simulink model "W02_surge_control"  (R2024b)
settings: Solver=ode4  StartTime=0  StopTime=T_final  FixedStep=h  RelTol=1e-3
StopFcn:
  | W02_plot;
values from neighbouring files (symbols this model uses):
  animate = 1    [W02_0_setup.m]
  aw_mode = 2    [W02_0_setup.m]
  beta_c = 0    [W02_0_setup.m]
  c_d = 0    [W02_0_setup.m]
  h = 0.02    [W02_0_setup.m]    (also in W02_1_build_pid.m = add_line(sys, [a; via; b]); W02_1_build_surge_control.m = Simulink.Annotation([m '/note']); W02_G_derivative_noise_and_kick.m = lab_fig('W02 G  kick', 1000, 420);  hold on; W02_G_noise_and_kick.m = lab_fig('W02 Exp 2-10c  kick', 1000, 420);  hold on)
  K_aw = 1/T_u    (= 0.907069384191)    [W02_0_setup.m]
  k_neg = cfg.k_neg    [W02_0_setup.m]
  k_pos = cfg.k_pos    [W02_0_setup.m]
  Kd = 0    [W02_0_setup.m]    (also in W02_E_integral.m = 4; W02_I_tuning_by_hand.m = 1)
  Ki = 192.38    [W02_0_setup.m]
  Kp = 102.00    (= 102)    [W02_0_setup.m]    (also in W02_D_derivative.m = 10; W02_E_integral.m = 10; W02_I_tuning_by_hand.m = 5*k)
  loop_closed = 1    [W02_0_setup.m]
  mp = 25    [W02_0_setup.m]
  n_max = cfg.n_max    [W02_0_setup.m]
  n_min = cfg.n_min    [W02_0_setup.m]
  Nf = 20    [W02_0_setup.m]    (also in W02_G_lowpass_filter.m = Nf(i))
  pid_mode = 0    [W02_0_setup.m]
  rp = [0.05 0 -0.35]'    [W02_0_setup.m]
  t_dn = 1e6    (= 1000000)    [W02_0_setup.m]
  t_up = 5    [W02_0_setup.m]
  u_d1 = 1.5    [W02_0_setup.m]
  u_d2 = 1.5    [W02_0_setup.m]
  V_c = 0    [W02_0_setup.m]
  x0 = zeros(12,1)    [W02_0_setup.m]
  X_hi = 2*k_pos*n_max^2    [W02_0_setup.m]    (also in W02_plot.m = 2*cfg.k_pos*cfg.n_max^2)
  X_lo = -2*k_neg*n_min^2    [W02_0_setup.m]    (also in W02_plot.m = -2*cfg.k_neg*cfg.n_min^2)
  X_open = 100    [W02_0_setup.m]
libraries: slpidlib x1
settings Model: Creator=admin  LastModifiedBy=admin
settings DataIOCC: ReturnWorkspaceOutputs=off

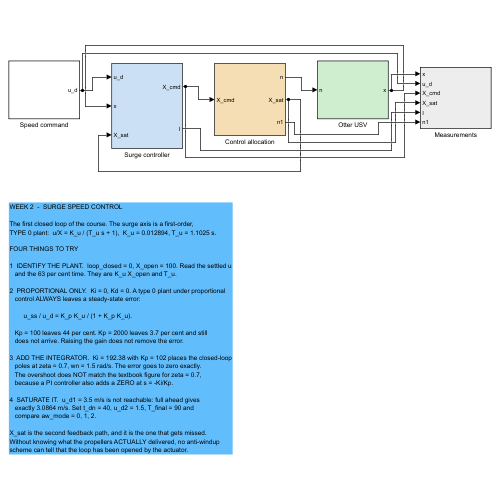
[thumbnail: Simulink's stored preview of the top-level diagram]
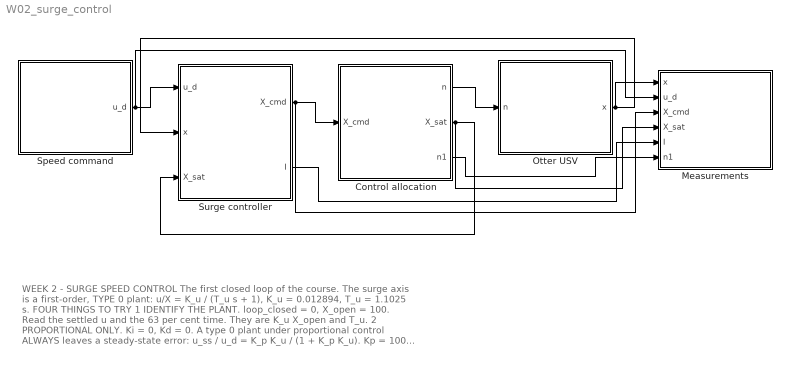
== system W02_surge_control ==
  note: WEEK 2  -  SURGE SPEED CONTROL
      |
      | The first closed loop of the course. The surge axis is a first-order,
      | TYPE 0 plant:  u/X = K_u / (T_u s + 1),  K_u = 0.012894, T_u = 1.1025 s.
      |
      | FOUR THINGS TO TRY
      |
      | 1  IDENTIFY THE PLANT.  loop_closed = 0, X_open = 100. Read the settled u
      |    and the 63 per cent time. They are K_u X_open and T_u.
      |
      | 2  PROPORTIONAL ONLY.  Ki = 0, Kd = 0. A type 0 plant under proportional
      |    control ALWAYS leaves a steady-state error:
      |
      |         u_ss / u_d = K_p K_u / (1 + K_p K_u).
      |
      |    Kp = 100 leaves 44 per cent. Kp = 2000 leaves 3.7 per cent and still
      |    does not arrive. Raising the gain does not remove the error.
      |
      | 3  ADD THE INTEGRATOR.  Ki = 192.38 with Kp = 102 places the closed-loop
      |    poles at zeta = 0.7, wn = 1.5 rad/s. The error goes to zero exactly.
      |    The overshoot does NOT match the textbook figure for zeta = 0.7,
      |    because a PI controller also adds a ZERO at s = -Ki/Kp.
      |
      | 4  SATURATE IT.  u_d1 = 3.5 m/s is not reachable: full ahead gives
      |    exactly 3.0864 m/s. Set t_dn = 40, u_d2 = 1.5, T_final = 90 and
      |    compare aw_mode = 0, 1, 2.
      |
      | X_sat is the second feedback path, and it is the one that gets missed.
      | Without knowing what the propellers ACTUALLY delivered, no anti-windup
      | scheme can tell that the loop has been opened by the actuator.
  Control allocation : Subsystem
  Measurements : Subsystem
  Otter USV : Subsystem
  Speed command : Subsystem
  Surge controller : Subsystem
  wires:
  Speed command/1(u_d) -> Surge controller/1(u_d), Measurements/2(u_d)
  Otter USV/1(x) -> Surge controller/2(x), Measurements/1(x)
  Control allocation/2(X_sat) -> Surge controller/3(X_sat), Measurements/4(X_sat)
  Surge controller/1(X_cmd) -> Control allocation/1(X_cmd), Measurements/3(X_cmd)
  Control allocation/1(n) -> Otter USV/1(n)
  Surge controller/2(I) -> Measurements/5(I)
  Control allocation/3(n1) -> Measurements/6(n1)

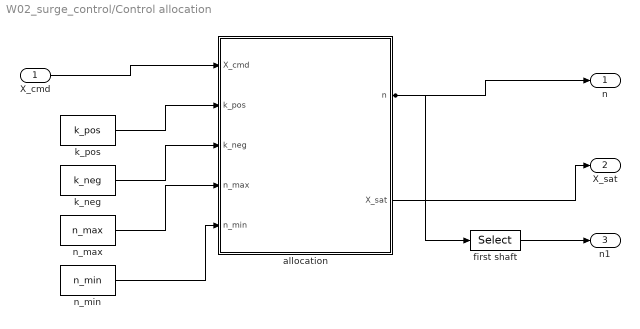
== system W02_surge_control/Control allocation ==
  X_cmd : Inport
  allocation : MATLAB Function  TreatAsAtomicUnit=on
  first shaft : Selector  InputPortWidth=2  IndexOptions=Index vector (dialog)  Indices=1  OutputSizes=1
  k_neg : Constant  Value=k_neg
  k_pos : Constant  Value=k_pos
  n_max : Constant  Value=n_max
  n_min : Constant  Value=n_min
  n : Outport
  X_sat : Outport  Port=2
  n1 : Outport  Port=3
  wires:
  X_cmd/1 -> allocation/1(X_cmd)
  k_pos/1 -> allocation/2(k_pos)
  k_neg/1 -> allocation/3(k_neg)
  n_max/1 -> allocation/4(n_max)
  n_min/1 -> allocation/5(n_min)
  allocation/1(n) -> n/1, first shaft/1
  first shaft/1 -> n1/1
  allocation/2(X_sat) -> X_sat/1

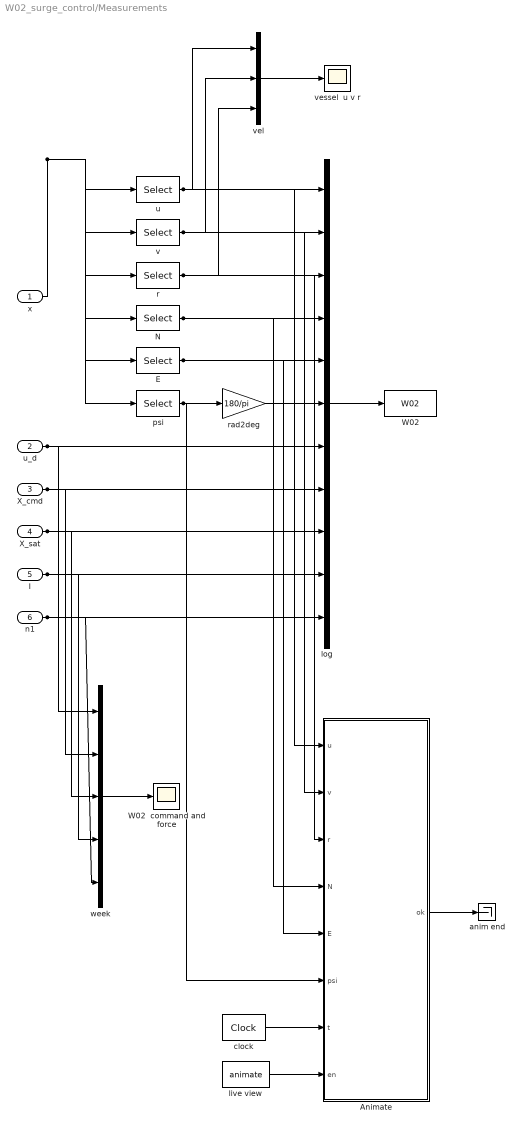
== system W02_surge_control/Measurements ==
  x : Inport
  u_d : Inport  Port=2
  X_cmd : Inport  Port=3
  X_sat : Inport  Port=4
  I : Inport  Port=5
  n1 : Inport  Port=6
  Animate : MATLAB Function  TreatAsAtomicUnit=on
  E : Selector  InputPortWidth=12  IndexOptions=Index vector (dialog)  Indices=8  OutputSizes=1
  N : Selector  InputPortWidth=12  IndexOptions=Index vector (dialog)  Indices=7  OutputSizes=1
  W02 : ToWorkspace  VariableName=W02  SaveFormat=Structure With Time  SampleTime=-1
  W02  command and force : Scope
  anim end : Terminator
  clock : DigitalClock  SampleTime=h
  live view : Constant  Value=animate
  log : Mux  Inputs=11
  psi : Selector  InputPortWidth=12  IndexOptions=Index vector (dialog)  Indices=12  OutputSizes=1
  r : Selector  InputPortWidth=12  IndexOptions=Index vector (dialog)  Indices=6  OutputSizes=1
  rad2deg : Gain  Gain=180/pi
  u : Selector  InputPortWidth=12  IndexOptions=Index vector (dialog)  Indices=1  OutputSizes=1
  v : Selector  InputPortWidth=12  IndexOptions=Index vector (dialog)  Indices=2  OutputSizes=1
  vel : Mux  Inputs=3
  vessel  u v r : Scope
  week : Mux  Inputs=5
  wires:
  x/1 -> u/1, v/1, r/1, N/1, E/1, psi/1
  log/1 -> W02/1
  psi/1 -> rad2deg/1, Animate/6(psi)
  u/1 -> log/1, vel/1, Animate/1(u)
  v/1 -> log/2, vel/2, Animate/2(v)
  r/1 -> log/3, vel/3, Animate/3(r)
  N/1 -> log/4, Animate/4(N)
  E/1 -> log/5, Animate/5(E)
  rad2deg/1 -> log/6
  u_d/1 -> log/7, week/1
  X_cmd/1 -> log/8, week/2
  X_sat/1 -> log/9, week/3
  I/1 -> log/10, week/4
  n1/1 -> log/11, week/5
  vel/1 -> vessel  u v r/1
  week/1 -> W02  command and force/1
  clock/1 -> Animate/7(t)
  live view/1 -> Animate/8(en)
  Animate/1(ok) -> anim end/1

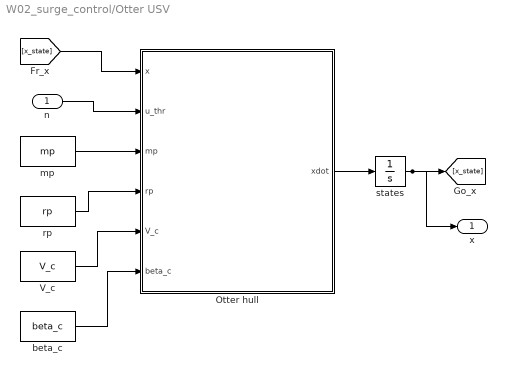
== system W02_surge_control/Otter USV ==
  n : Inport
  Otter hull : MATLAB Function  TreatAsAtomicUnit=on
  V_c : Constant  Value=V_c
  beta_c : Constant  Value=beta_c
  mp : Constant  Value=mp
  rp : Constant  Value=rp
  states : Integrator  InitialCondition=x0
  x : Outport
  wires:
  states/1 -> [x_state], x/1
  Otter hull/1(xdot) -> states/1
  beta_c/1 -> Otter hull/6(beta_c)
  [x_state] -> Otter hull/1(x)
  rp/1 -> Otter hull/4(rp)
  n/1 -> Otter hull/2(u_thr)
  mp/1 -> Otter hull/3(mp)
  V_c/1 -> Otter hull/5(V_c)

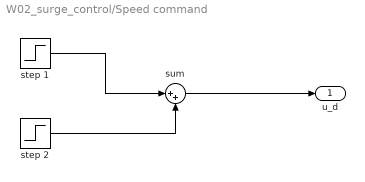
== system W02_surge_control/Speed command ==
  step 1 : Step  Time=t_up  After=u_d1  SampleTime=0
  step 2 : Step  Time=t_dn  After=u_d2 - u_d1  SampleTime=0
  sum : Sum  Inputs=|++
  u_d : Outport
  wires:
  step 1/1 -> sum/1
  step 2/1 -> sum/2
  sum/1 -> u_d/1

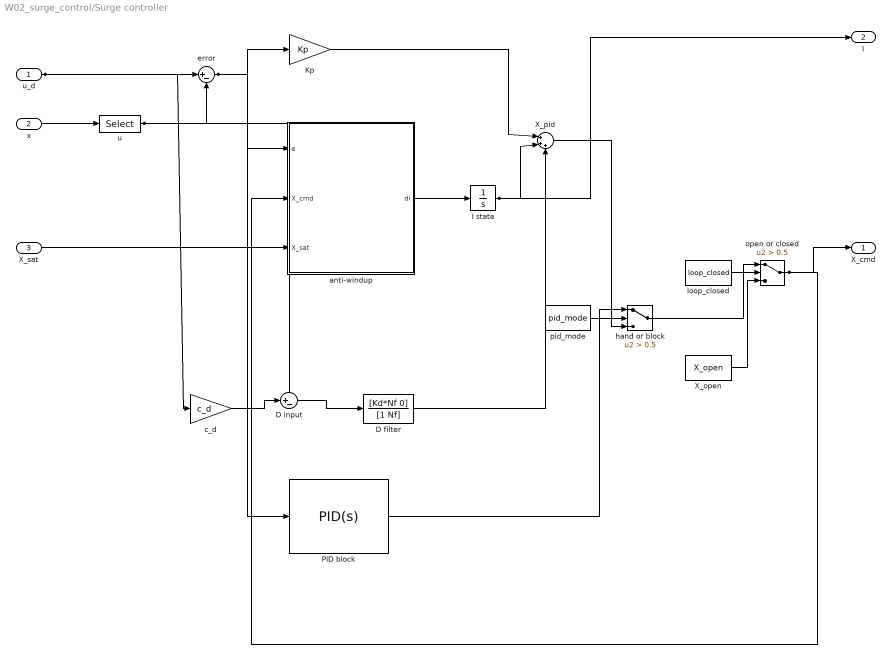
== system W02_surge_control/Surge controller ==
  u_d : Inport
  x : Inport  Port=2
  X_sat : Inport  Port=3
  D filter : TransferFcn  Numerator=[Kd*Nf 0]  Denominator=[1 Nf]
  D input : Sum  Inputs=|+-
  I state : Integrator
  Kp : Gain  Gain=Kp
  PID block : slpidlib/PID Controller  Controller=PID  Form=Parallel  TimeDomain=Continuous-time  UseExternalTs=off  SampleTime=-1  IntegratorMethod=Forward Euler  FilterMethod=Forward Euler  ControllerParametersSource=internal  P=Kp  I=Ki  UseKiTs=off  D=Kd  UseExternalDerivativeSource=off  N=Nf  UseFilter=on  TunerSelectOption=Transfer Function Based (PID Tuner App)  InitialConditionSource=internal  InitialConditionForIntegrator=0  InitialConditionForFilter=0  DifferentiatorICPrevScaledInput=0  ExternalReset=none  TrackingMode=off  Kt=1  LimitOutput=on  SatLimitsSource=internal  UpperSaturationLimit=X_hi  LowerSaturationLimit=X_lo  LinearizeAsGain=on  AntiWindupMode=back-calculation  Kb=K_aw  LimitIntegrator=off  UpperIntegratorSaturationLimit=inf  LowerIntegratorSaturationLimit=-inf  POutMin=[]  POutMax=[]  IOutMin=[]  IOutMax=[]  DOutMin=[]  DOutMax=[]  NOutMin=[]  NOutMax=[]  SumOutMin=[]  SumOutMax=[]  SaturationOutMin=[]  SaturationOutMax=[]  PParamMin=[]  PParamMax=[]  IParamMin=[]  IParamMax=[]  DParamMin=[]  DParamMax=[]  NParamMin=[]  NParamMax=[]  KbParamMin=[]  KbParamMax=[]  KtParamMin=[]  KtParamMax=[]  KbOutMin=[]  KbOutMax=[]  KtOutMin=[]  KtOutMax=[]  IntegratorOutMin=[]  IntegratorOutMax=[]  FilterOutMin=[]  FilterOutMax=[]  SumI1OutMin=[]  SumI1OutMax=[]  SumI2OutMin=[]  SumI2OutMax=[]  SumI3OutMin=[]  SumI3OutMax=[]  SumI4OutMin=[]  SumI4OutMax=[]  SumDOutMin=[]  SumDOutMax=[]  DifferentiatorOutMin=[]  DifferentiatorOutMax=[]  FilterDiffOutCoefMin=[]  FilterDiffOutCoefMax=[]  ReciprocalOutMin=[]  ReciprocalOutMax=[]  SumDenOutMin=[]  SumDenOutMax=[]  SumNumOutMin=[]  SumNumOutMax=[]  DivideOutMin=[]  DivideOutMax=[]  UdiffTsProdOutMin=[]  UdiffTsProdOutMax=[]  NTsProdOutMin=[]  NTsProdOutMax=[]  UintegralTsProdOutMin=[]  UintegralTsProdOutMax=[]  UngainTsProdOutMin=[]  UngainTsProdOutMax=[]  ClampingZeroOutDataTypeStr=Inherit: Inherit via back propagation  ClampingZeroOutMin=[]  ClampingZeroOutMax=[]  FilterDenConstantOutDataTypeStr=Inherit: Inherit via back propagation  FilterDenConstantOutMin=[]  FilterDenConstantOutMax=[]  PCopyOutDataTypeStr=Inherit: Inherit via back propagation  PCopyOutMin=[]  PCopyOutMax=[]  NCopyOutDataTypeStr=Inherit: Inherit via back propagation  NCopyOutMin=[]  NCopyOutMax=[]  IntegratorContinuousStateAttributes=''  IntegratorStateMustResolveToSignalObject=off  IntegratorRTWStateStorageClass=Auto  FilterContinuousStateAttributes=''  FilterStateMustResolveToSignalObject=off  FilterRTWStateStorageClass=Auto  ParallelPVariant=InternalParameters  IdealPVariant=Disabled  IVariant=InternalParameters  DVariant=InternalParameters  IntegratorVariant=Continuous  SatVariant=Enabled  AWVariant=BackCalculation  PCopyVariant=Disabled  TRVariant=Disabled  FdbkBlocksVariant=Forward  IdealPFdbkVariant=Disabled  SatFdbkVariant=Disabled  DerivativeFilterVariant=ContFilter  NVariant=InternalParameters  NCopyVariant=Disabled  FilterICVariant=InternalICsFilter  IntegratorICVariant=InternalICs  ExternalResetVariant=Disabled  TRSumVariant=Passthrough  SumFdbkVariant=Disabled  SumVariant=Sum_PID  TsampFilterVariant=InternalTs  TsampNgainVariant=Passthrough  TsampIntegralVariant=Disabled_SignalSpec  ExternalSaturationOutDataTypeStr=Inherit: Same as second input  DerivativeSourceVariant=ErrorSignal  PreIntVariant=InternalPreInt
  X_open : Constant  Value=X_open
  X_pid : Sum  Inputs=|+++
  anti-windup : Subsystem
  c_d : Gain  Gain=c_d
  error : Sum  Inputs=|+-
  hand or block : Switch  Criteria=u2 > Threshold  Threshold=0.5  SaturateOnIntegerOverflow=off  InputSameDT=off
  loop_closed : Constant  Value=loop_closed
  open or closed : Switch  Criteria=u2 > Threshold  Threshold=0.5  SaturateOnIntegerOverflow=off  InputSameDT=off
  pid_mode : Constant  Value=pid_mode
  u : Selector  InputPortWidth=12  IndexOptions=Index vector (dialog)  Indices=1  OutputSizes=1
  X_cmd : Outport
  I : Outport  Port=2
  wires:
  x/1 -> u/1
  u_d/1 -> error/1, c_d/1
  u/1 -> error/2, D input/2
  error/1 -> Kp/1, anti-windup/1(e), PID block/1
  X_sat/1 -> anti-windup/3(X_sat)
  anti-windup/1(di) -> I state/1
  c_d/1 -> D input/1
  D input/1 -> D filter/1
  Kp/1 -> X_pid/1
  I state/1 -> X_pid/2, I/1
  D filter/1 -> X_pid/3
  pid_mode/1 -> hand or block/2
  PID block/1 -> hand or block/1
  X_pid/1 -> hand or block/3
  loop_closed/1 -> open or closed/2
  X_open/1 -> open or closed/3
  hand or block/1 -> open or closed/1
  open or closed/1 -> X_cmd/1, anti-windup/2(X_cmd)

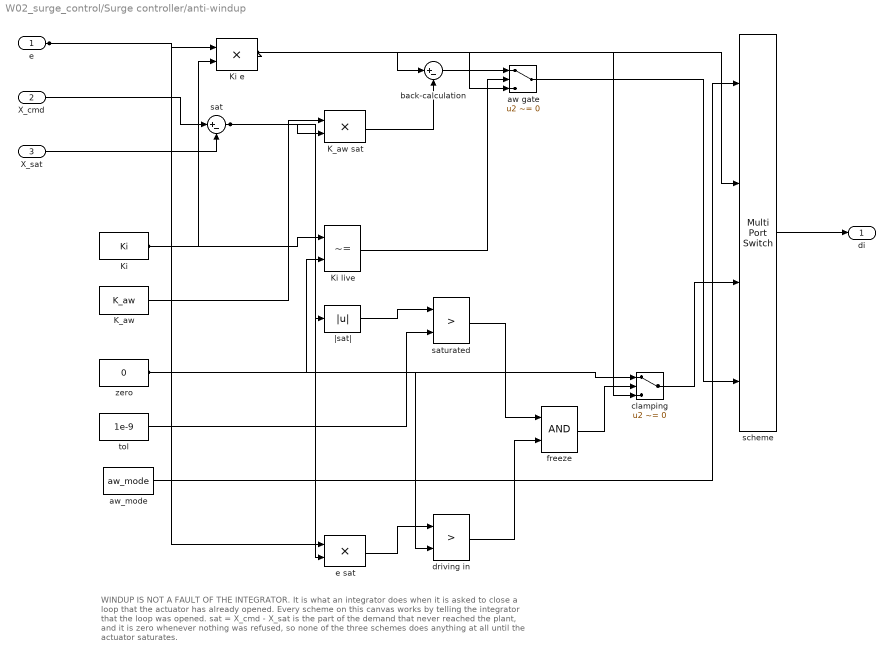
== system W02_surge_control/Surge controller/anti-windup ==
  note: WINDUP IS NOT A FAULT OF THE INTEGRATOR.
      | It is what an integrator does when it is asked to close a loop that the actuator has already opened.
      | Every scheme on this canvas works by telling the integrator that the loop was opened. sat = X_cmd - X_sat
      | is the part of the demand that never reached the plant, and it is zero whenever nothing was refused, so
      | none of the three schemes does anything at all until the actuator saturates.
  e : Inport
  X_cmd : Inport  Port=2
  X_sat : Inport  Port=3
  K_aw : Constant  Value=K_aw
  K_aw sat : Product
  Ki : Constant  Value=Ki
  Ki e : Product
  Ki live : RelationalOperator  Operator=~=  OutDataTypeStr=boolean  RndMeth=Simplest  InputSameDT=off
  aw gate : Switch  Criteria=u2 ~= 0  SaturateOnIntegerOverflow=off  InputSameDT=off
  aw_mode : Constant  Value=aw_mode
  back-calculation : Sum  Inputs=|+-
  clamping : Switch  Criteria=u2 ~= 0  SaturateOnIntegerOverflow=off  InputSameDT=off
  driving in : RelationalOperator  Operator=>  OutDataTypeStr=boolean  RndMeth=Simplest  InputSameDT=off
  e sat : Product
  freeze : Logic  AllPortsSameDT=off  OutDataTypeStr=boolean
  sat : Sum  Inputs=|+-
  saturated : RelationalOperator  Operator=>  OutDataTypeStr=boolean  RndMeth=Simplest  InputSameDT=off
  scheme : MultiPortSwitch  DataPortOrder=Zero-based contiguous  zeroidx=on  SaturateOnIntegerOverflow=off  InputSameDT=off
  tol : Constant  Value=1e-9
  zero : Constant  Value=0
  |sat| : Abs  SaturateOnIntegerOverflow=off
  di : Outport
  wires:
  X_cmd/1 -> sat/1
  X_sat/1 -> sat/2
  e/1 -> Ki e/1, e sat/1
  Ki/1 -> Ki e/2, Ki live/1
  K_aw/1 -> K_aw sat/1
  sat/1 -> K_aw sat/2, |sat|/1, e sat/2
  Ki e/1 -> back-calculation/1, aw gate/3, clamping/3, scheme/2
  K_aw sat/1 -> back-calculation/2
  zero/1 -> Ki live/2, driving in/2, clamping/1
  back-calculation/1 -> aw gate/1
  Ki live/1 -> aw gate/2
  |sat|/1 -> saturated/1
  tol/1 -> saturated/2
  e sat/1 -> driving in/1
  saturated/1 -> freeze/1
  driving in/1 -> freeze/2
  freeze/1 -> clamping/2
  aw_mode/1 -> scheme/1
  clamping/1 -> scheme/3
  aw gate/1 -> scheme/4
  scheme/1 -> di/1

== matlab function W02_surge_control/Otter USV/Otter hull ==
  data: x input; xdot output double size=[12 1]; u_thr input; mp input; rp input; V_c input; beta_c input
function xdot = otter_hull(x, u_thr, mp, rp, V_c, beta_c)
% Fossen's otter.m, called unchanged from Tools/MSS/VESSELS.
%
%   x       12 states, fed back from the integrator
%   u_thr   propeller shaft speeds [rad/s]
%
% otter.m is not written for code generation, so the call is extrinsic and
% xdot has to be pre-sized for Simulink to know the output width.
coder.extrinsic('otter');

xdot = zeros(12,1);
xdot = otter(x, u_thr, mp, rp, V_c, beta_c);
end

== matlab function W02_surge_control/Control allocation/allocation ==
  data: X_cmd input; n output double size=[2 1]; k_pos input; k_neg input; n_max input; n_min input; X_sat output
function [n, X_sat] = allocation(X_cmd, k_pos, k_neg, n_max, n_min)
%#codegen
% Demanded surge force to shaft speed, and back again.
%
% The demand is split equally between the two propellers, because nothing in
% a pure surge command distinguishes them. Inverting T = k n|n| gives
%
%     n = sign(T) sqrt(|T| / k)
%
% X_sat is what the propellers ACTUALLY produce after saturation. Without it
% the controller cannot know that the loop has been opened by the actuator,
% and no anti-windup scheme can work.
T = X_cmd / 2;
if T >= 0
    ni =  sqrt( T / k_pos);
else
    ni = -sqrt(-T / k_neg);
end
ni = min(max(ni, n_min), n_max);
n = [ni; ni];
if ni >= 0
    X_sat = 2 * k_pos * ni * abs(ni);
else
    X_sat = 2 * k_neg * ni * abs(ni);
end
end

== matlab function W02_surge_control/Measurements/Animate ==
  data: u input; ok output; v input; r input; N input; E input; psi input; t input; en input
function ok = Animate(u, v, r, N, E, psi, t, en)
%#codegen
% Live view of the vessel while the model runs.
%
% A MATLAB Function block cannot plot, so the drawing function is declared
% extrinsic: Simulink calls plain MATLAB rather than generating code for it.
% Set animate = 0 in the setup script to switch the live view off.
%
% psi arrives in RADIANS and r in rad/s - the units otter.m works in. The
% wrapper converts them for display, in one place, so no two figures in the
% course can disagree about what a degree is.
coder.extrinsic('W02_animate');
ok = 1;
if en > 0.5
    W02_animate(u, v, r, N, E, psi, t);
end
end
